simulink model "simu3"  (R2020b)
settings: Solver=VariableStepAuto  StartTime=0.0  StopTime=Ttt  MaxStep=0.01  RelTol=1e-3
values from neighbouring files (symbols this model uses):
  kp = t_kp(i)    [lab3.m]    (also in lab3_2.m; lab3_4.m = 2.22; lab3_pi.m; test2.m = 1)
settings Model: Creator=pkubo  LastModifiedBy=pkubo
settings DataIOCC: ReturnWorkspaceOutputs=off

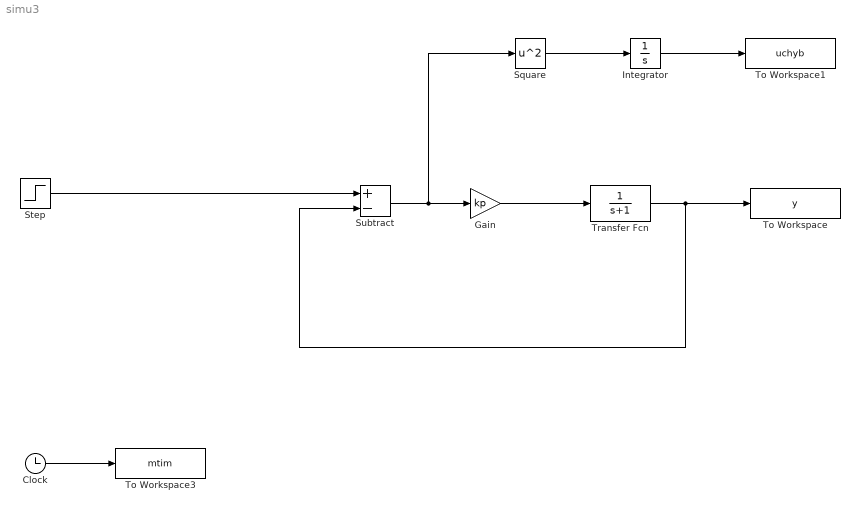
== system simu3 ==
  Clock : Clock
  Gain : Gain  Gain=kp
  Integrator : Integrator
  Square : Math  Operator=square  SignedPower=on  RndMeth=Zero  SaturateOnIntegerOverflow=on
  Step : Step  SampleTime=0
  Subtract : Sum  Inputs=+-
  To Workspace : ToWorkspace  VariableName=y  SampleTime=-1
  To Workspace1 : ToWorkspace  VariableName=uchyb  SampleTime=-1
  To Workspace3 : ToWorkspace  VariableName=mtim  SampleTime=-1
  Transfer Fcn : TransferFcn  Denominator=[1 1]
  wires:
  Transfer Fcn/1 -> Subtract/2, To Workspace/1
  Clock/1 -> To Workspace3/1
  Gain/1 -> Transfer Fcn/1
  Step/1 -> Subtract/1
  Integrator/1 -> To Workspace1/1
  Square/1 -> Integrator/1
  Subtract/1 -> Square/1, Gain/1
